simulink model "Production"  (R2025b)
settings: Solver=VariableStepAuto  StartTime=0.0  StopTime=105600  RelTol=1e-3
undefined symbols (not defined in the file or in its folder): m, n
(part 2 of 2)

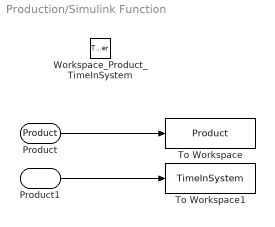
== system Production/Simulink Function ==
  Workspace_Product_TimeInSystem : TriggerPort  TriggerType=function-call  IsSimulinkFunction=on  FunctionName=Workspace_Product_TimeInSystem  FunctionVisibility=scoped  VariantControl=(inherit)
  To Workspace : ToWorkspace  VariableName=Product  SaveFormat=Timeseries  SampleTime=-1
  To Workspace1 : ToWorkspace  VariableName=TimeInSystem  SaveFormat=Timeseries  SampleTime=-1
  Product : ArgIn  DisableCoverage=on  ArgumentName=Product
  Product1 : ArgIn  DisableCoverage=on  Port=2  ArgumentName=TimeInSystem
  wires:
  Product/1 -> To Workspace/1
  Product1/1 -> To Workspace1/1

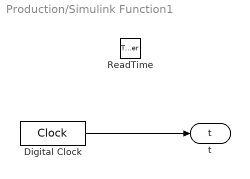
== system Production/Simulink Function1 ==
  ReadTime : TriggerPort  TriggerType=function-call  IsSimulinkFunction=on  FunctionName=ReadTime  FunctionVisibility=scoped  VariantControl=(inherit)
  Digital Clock : DigitalClock  SampleTime=-1
  t : ArgOut  DisableCoverage=on  ArgumentName=t
  wires:
  Digital Clock/1 -> t/1

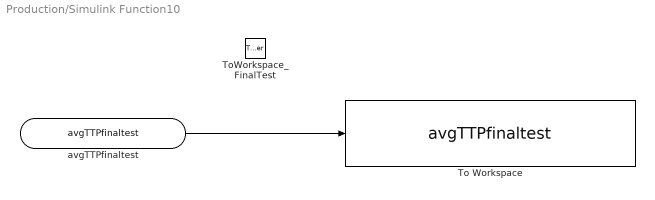
== system Production/Simulink Function10 ==
  ToWorkspace_FinalTest : TriggerPort  TriggerType=function-call  IsSimulinkFunction=on  FunctionName=ToWorkspace_FinalTest  FunctionVisibility=scoped  VariantControl=(inherit)
  To Workspace : ToWorkspace  VariableName=avgTTPfinaltest  SaveFormat=Timeseries  SampleTime=-1
  avgTTPfinaltest : ArgIn  ArgumentName=avgTTPfinaltest
  wires:
  avgTTPfinaltest/1 -> To Workspace/1

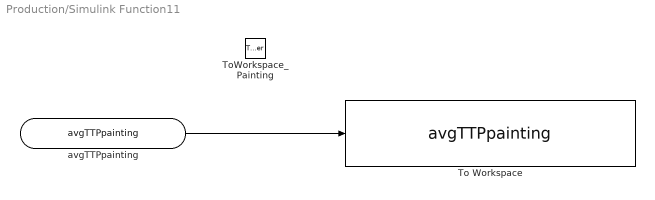
== system Production/Simulink Function11 ==
  ToWorkspace_Painting : TriggerPort  TriggerType=function-call  IsSimulinkFunction=on  FunctionName=ToWorkspace_Painting  FunctionVisibility=scoped  VariantControl=(inherit)
  To Workspace : ToWorkspace  VariableName=avgTTPpainting  SaveFormat=Timeseries  SampleTime=-1
  avgTTPpainting : ArgIn  ArgumentName=avgTTPpainting
  wires:
  avgTTPpainting/1 -> To Workspace/1

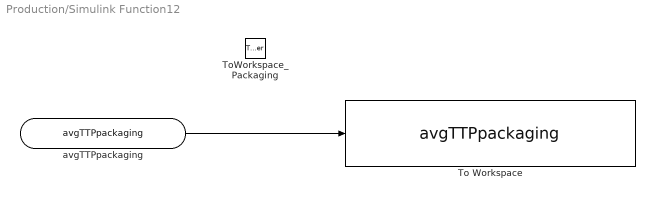
== system Production/Simulink Function12 ==
  ToWorkspace_Packaging : TriggerPort  TriggerType=function-call  IsSimulinkFunction=on  FunctionName=ToWorkspace_Packaging  FunctionVisibility=scoped  VariantControl=(inherit)
  To Workspace : ToWorkspace  VariableName=avgTTPpackaging  SaveFormat=Timeseries  SampleTime=-1
  avgTTPpackaging : ArgIn  ArgumentName=avgTTPpackaging
  wires:
  avgTTPpackaging/1 -> To Workspace/1

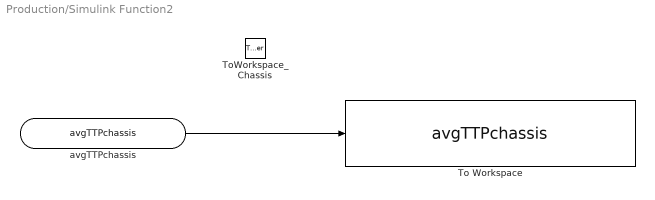
== system Production/Simulink Function2 ==
  ToWorkspace_Chassis : TriggerPort  TriggerType=function-call  IsSimulinkFunction=on  FunctionName=ToWorkspace_Chassis  FunctionVisibility=scoped  VariantControl=(inherit)
  To Workspace : ToWorkspace  VariableName=avgTTPchassis  SaveFormat=Timeseries  SampleTime=-1
  avgTTPchassis : ArgIn  ArgumentName=avgTTPchassis
  wires:
  avgTTPchassis/1 -> To Workspace/1

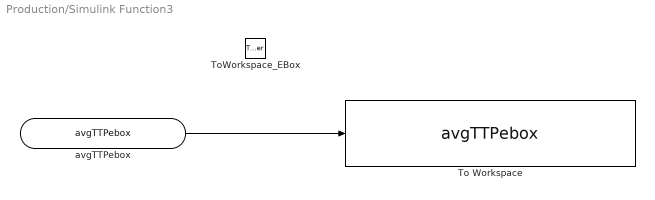
== system Production/Simulink Function3 ==
  ToWorkspace_EBox : TriggerPort  TriggerType=function-call  IsSimulinkFunction=on  FunctionName=ToWorkspace_EBox  FunctionVisibility=scoped  VariantControl=(inherit)
  To Workspace : ToWorkspace  VariableName=avgTTPebox  SaveFormat=Timeseries  SampleTime=-1
  avgTTPebox : ArgIn  ArgumentName=avgTTPebox
  wires:
  avgTTPebox/1 -> To Workspace/1

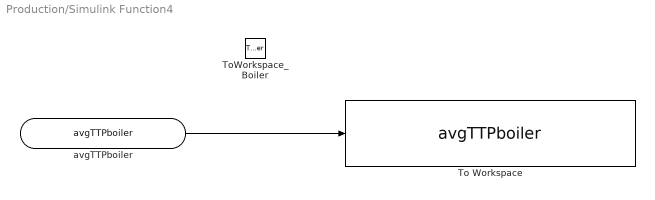
== system Production/Simulink Function4 ==
  ToWorkspace_Boiler : TriggerPort  TriggerType=function-call  IsSimulinkFunction=on  FunctionName=ToWorkspace_Boiler  FunctionVisibility=scoped  VariantControl=(inherit)
  To Workspace : ToWorkspace  VariableName=avgTTPboiler  SaveFormat=Timeseries  SampleTime=-1
  avgTTPboiler : ArgIn  ArgumentName=avgTTPboiler
  wires:
  avgTTPboiler/1 -> To Workspace/1

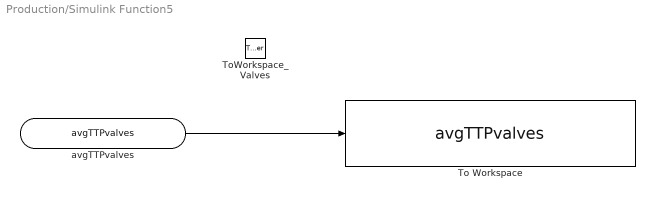
== system Production/Simulink Function5 ==
  ToWorkspace_Valves : TriggerPort  TriggerType=function-call  IsSimulinkFunction=on  FunctionName=ToWorkspace_Valves  FunctionVisibility=scoped  VariantControl=(inherit)
  To Workspace : ToWorkspace  VariableName=avgTTPvalves  SaveFormat=Timeseries  SampleTime=-1
  avgTTPvalves : ArgIn  ArgumentName=avgTTPvalves
  wires:
  avgTTPvalves/1 -> To Workspace/1

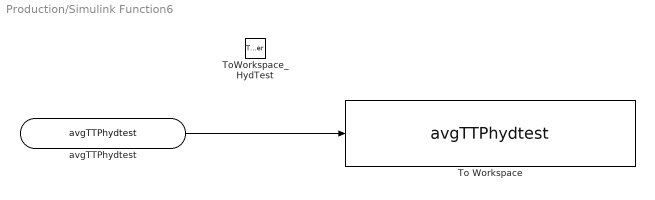
== system Production/Simulink Function6 ==
  ToWorkspace_HydTest : TriggerPort  TriggerType=function-call  IsSimulinkFunction=on  FunctionName=ToWorkspace_HydTest  FunctionVisibility=scoped  VariantControl=(inherit)
  To Workspace : ToWorkspace  VariableName=avgTTPhydtest  SaveFormat=Timeseries  SampleTime=-1
  avgTTPhydtest : ArgIn  ArgumentName=avgTTPhydtest
  wires:
  avgTTPhydtest/1 -> To Workspace/1

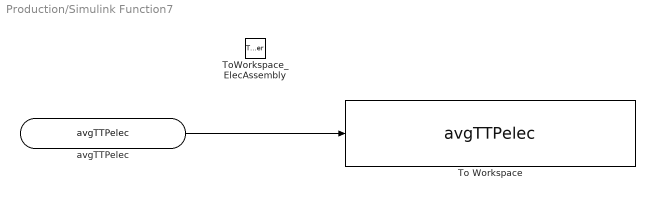
== system Production/Simulink Function7 ==
  ToWorkspace_ElecAssembly : TriggerPort  TriggerType=function-call  IsSimulinkFunction=on  FunctionName=ToWorkspace_ElecAssembly  FunctionVisibility=scoped  VariantControl=(inherit)
  To Workspace : ToWorkspace  VariableName=avgTTPelec  SaveFormat=Timeseries  SampleTime=-1
  avgTTPelec : ArgIn  ArgumentName=avgTTPelec
  wires:
  avgTTPelec/1 -> To Workspace/1

== system Production/Simulink Function8 ==
  ToWorkspace_ElecTest : TriggerPort  TriggerType=function-call  IsSimulinkFunction=on  FunctionName=ToWorkspace_ElecTest  FunctionVisibility=scoped  VariantControl=(inherit)
  To Workspace : ToWorkspace  VariableName=avgTTPelectest  SaveFormat=Timeseries  SampleTime=-1
  avgTTPelectest : ArgIn  ArgumentName=avgTTPelectest
  wires:
  avgTTPelectest/1 -> To Workspace/1

== system Production/Simulink Function9 ==
  ToWorkspace_Components : TriggerPort  TriggerType=function-call  IsSimulinkFunction=on  FunctionName=ToWorkspace_Components  FunctionVisibility=scoped  VariantControl=(inherit)
  To Workspace : ToWorkspace  VariableName=avgTTPcomponents  SaveFormat=Timeseries  SampleTime=-1
  avgTTPcomponents : ArgIn  ArgumentName=avgTTPcomponents
  wires:
  avgTTPcomponents/1 -> To Workspace/1
